simulink model "corde"  (R2019b)
settings: Solver=VariableStepAuto  StartTime=0.0  StopTime=10  RelTol=1e-3
libraries: dspsrcs4 x1
settings Model: Creator=jeanz  LastModifiedBy=jeanz

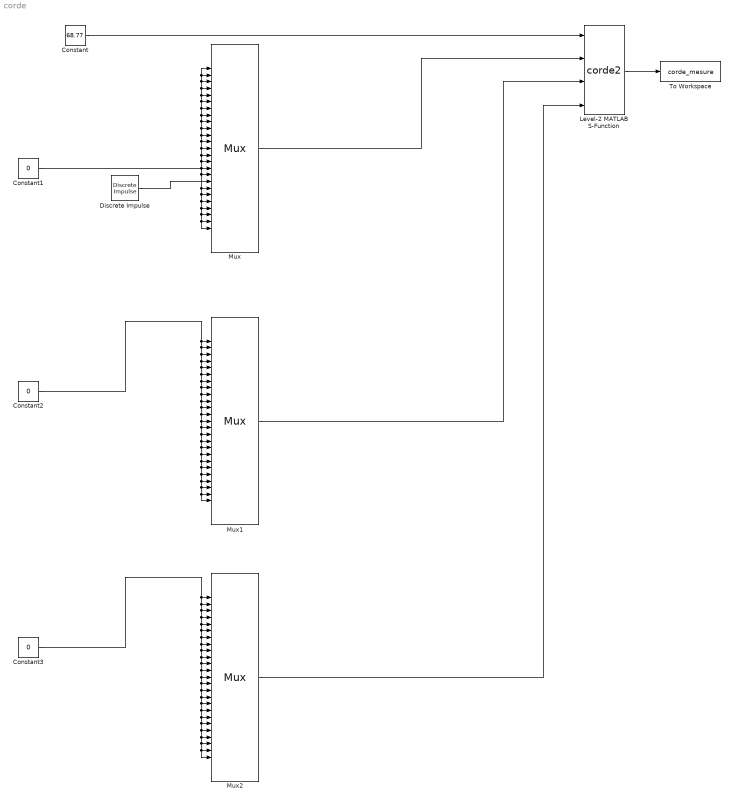
== system corde ==
  Constant : Constant  Value=68.77
  Constant1 : Constant  Value=0
  Constant2 : Constant  Value=0
  Constant3 : Constant  Value=0
  Discrete Impulse : dspsrcs4/Discrete  Impulse  Delay=1  SampleTime=0.01  FrameSample=1  OutputFrames=off  dataType=double  isSigned=on  wordLen=16  udDataType=sfix(16)  fracBitsMode=Best precision  numFracBits=15  OutDataTypeStr=double  LastOutDataTypeStr=double
  Level-2 MATLAB S-Function : M-S-Function  FunctionName=corde2  Parameters=0.00325, 0.44, 0, 25
  Mux : Mux  Inputs=25
  Mux1 : Mux  Inputs=25
  Mux2 : Mux  Inputs=25
  To Workspace : ToWorkspace  VariableName=corde_mesure  SaveFormat=Timeseries  SampleTime=0.0005
  wires:
  Constant/1 -> Level-2 MATLAB S-Function/1
  Constant1/1 -> Mux/15, Mux/13, Mux/12, Mux/11, Mux/10, Mux/1, Mux/2, Mux/3, Mux/4, Mux/5, Mux/6, Mux/7, Mux/8, Mux/9, Mux/14, Mux/25, Mux/24, Mux/23, Mux/22, Mux/21, Mux/20, Mux/19, Mux/17, Mux/16
  Mux/1 -> Level-2 MATLAB S-Function/2
  Constant2/1 -> Mux1/1, Mux1/2, Mux1/3, Mux1/4, Mux1/6, Mux1/25, Mux1/24, Mux1/23, Mux1/22, Mux1/21, Mux1/20, Mux1/19, Mux1/18, Mux1/17, Mux1/16, Mux1/15, Mux1/14, Mux1/13, Mux1/12, Mux1/11, Mux1/10, Mux1/9, Mux1/8, Mux1/7, Mux1/5
  Mux1/1 -> Level-2 MATLAB S-Function/3
  Constant3/1 -> Mux2/1, Mux2/2, Mux2/3, Mux2/4, Mux2/6, Mux2/25, Mux2/24, Mux2/23, Mux2/22, Mux2/21, Mux2/20, Mux2/19, Mux2/18, Mux2/17, Mux2/16, Mux2/15, Mux2/14, Mux2/13, Mux2/12, Mux2/11, Mux2/10, Mux2/9, Mux2/8, Mux2/7, Mux2/5
  Mux2/1 -> Level-2 MATLAB S-Function/4
  Level-2 MATLAB S-Function/1 -> To Workspace/1
  Discrete Impulse/1 -> Mux/18
